simulink model "sldemo_dblcart1"  (R2012b)
settings: Solver=ode23  SolverMode=SingleTasking  StartTime=0  StopTime=250  MaxStep=0.1  RelTol=1e-3  AbsTol=1e-6
PostLoadFcn:
  | crtanim2([],[],[],0,1);
model workspace (MAT data in the model file):
  ka = 1
  m1 = 1
  m2 = 1
  K = [3.08189689488 2.48269889228 0.0803807652926 3.18658131281]
  ae = [0  1  -31.4507297013  0; -1  0  44.8536687603  0; 0  0  -46.6599405981  1; 1  0  -89.5750283103  0]
  be = [0  31.4507297013; 1  -43.8536687603; 0  46.6599405981; 0  88.5750283103]
  ce = [1  0  0  0; 0  1  0  0; 0  0  1  0; 0  0  0  1]
  de = [0  0; 0  0; 0  0; 0  0]
  xSpr = [0; 0.4; 0.8; 1.6; 2.4; 3.2; 3.6; 4]
  xBx1 = [0; 0; -2; -2; 0]
  xBx2 = [0; 2; 2; 0; 0]
Description:
  | Double Spring Mass System
  | 
  | This example shows how to model a double spring-mass-damper system with a periodically
  | varying forcing function.  Associated with the example is an animation function
  | that will automatically open a figure window and display to it. In this system,
  | the only sensor is attached to the mass on the left, and the actuator is
  | attached to the mass on the left. State estimation and LQR control are used.
settings Model: ExtModeAutoUpdateStatusClock=off  Creator=The MathWorks Inc.  LastModifiedBy=re40768
settings DataIOCC: ExternalInput=[]  InitialState=[]  LimitDataPoints=off  SignalLoggingSaveFormat=ModelDataLogs  SaveOutput=off  SaveTime=off
settings OptimizationCC: BlockReduction=off  BooleanDataType=off  InlineInvariantSignals=on  InitFltsAndDblsToZero=on  BufferReusableBoundary=off
settings DebuggingCC: SaveWithParameterizedLinksMsg=none  SignalResolutionControl=TryResolveAllWithWarning  SolverPrmCheckMsg=none  MultiTaskDSMMsg=warning  MultiTaskCondExecSysMsg=none  FcnCallInpInsideContextMsg=UseLocalSettings  BusObjectLabelMismatch=none
settings HardwareCC: TargetUnknown=on
settings RTWCC: IncludeERTFirstTime=on
settings GRTTargetCC: TargetFcnLib=ansi_tfl_tmw.mat  CombineOutputUpdateFcns=off  GRTInterface=on

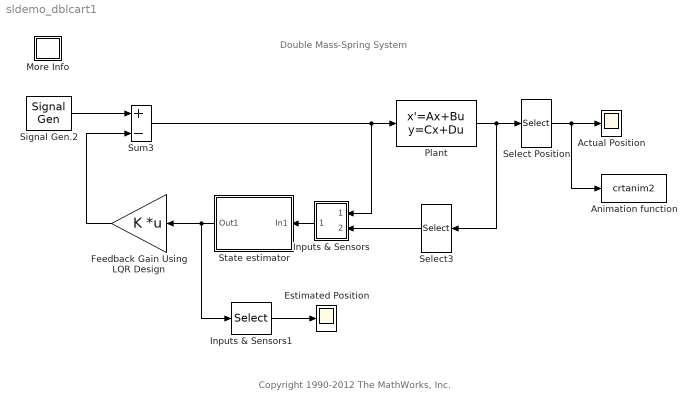
== system sldemo_dblcart1 ==
  note: Double Mass-Spring System
  note: Copyright 1990-2012 The MathWorks, Inc.
  Actual Position : Scope
      settings: TickLabels=on  TimeRange=40.000000
  Animation function : S-Function  FunctionName=crtanim2  Parameters=0.1  EnableBusSupport=off
      settings: DeleteFcn=shh = get(0,'ShowHiddenHandles');set(0,'ShowHiddenHandles','on');if ~isempty(findobj('type','figure','name','dblcart1 Animation'));close('dblcart1 Animation'); end;set(0,'ShowHiddenHandles',shh);
  Estimated Position : Scope
      settings: TickLabels=on  TimeRange=40.000000
  Feedback Gain Using LQR Design : Gain  Gain=K  Multiplication=Matrix(K*u) (u vector)
  Inputs & Sensors : Subsystem
  Inputs & Sensors1 : Selector  InputPortWidth=4  IndexOptions=Index vector (dialog)  Indices=[1 3]  OutputSizes=1
  More Info : Subsystem
      settings: OpenFcn=showdemo(bdroot(gcs))
      mask Display: disp('?')
  Plant : StateSpace  A=[0 1 0 0; -ka/m1 0 ka/m1 0; 0 0 0 1;ka/m2 0 -ka/m2 0]  B=[0; 1; 0; 0]  C=[1 0 0 0;0 0 1 0;0 0 1 0]  D=zeros(3,1)
  Select Position : Selector  InputPortWidth=3  IndexOptions=Index vector (dialog)  Indices=[1,2]  OutputSizes=1
  Select3 : Selector  InputPortWidth=3  IndexOptions=Index vector (dialog)  Indices=3  OutputSizes=1
  Signal Gen.2 : SignalGenerator  WaveForm=square  Amplitude=15  Frequency=0.300000  Units=rad/sec
  State estimator : Subsystem
  Sum3 : Sum  Inputs=+-  SaturateOnIntegerOverflow=on  InputSameDT=on  OutDataTypeStr=Inherit: Same as first input
  wires:
  State estimator/1(Out1) -> Inputs & Sensors1/1, Feedback Gain Using LQR Design/1
  Inputs & Sensors/1(Out1) -> State estimator/1(In1)
  Sum3/1 -> Inputs & Sensors/1(In1), Plant/1
  Feedback Gain Using LQR Design/1 -> Sum3/2
  Plant/1 -> Select3/1, Select Position/1
  Signal Gen.2/1 -> Sum3/1
  Inputs & Sensors1/1 -> Estimated Position/1
  Select3/1 -> Inputs & Sensors/2(In2)
  Select Position/1 -> Actual Position/1, Animation function/1

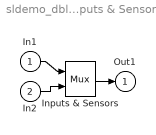
== system sldemo_dblcart1/Inputs & Sensors ==
  In1 : Inport
  In2 : Inport  Port=2
  Inputs & Sensors : Mux  Inputs=2
  Out1 : Outport  InitialOutput=0
  wires:
  In1/1 -> Inputs & Sensors/1
  In2/1 -> Inputs & Sensors/2
  Inputs & Sensors/1 -> Out1/1

== system sldemo_dblcart1/More Info ==

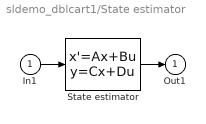
== system sldemo_dblcart1/State estimator ==
  In1 : Inport
  State estimator : StateSpace  A=ae  B=be  C=ce  D=de
  Out1 : Outport  InitialOutput=0
  wires:
  In1/1 -> State estimator/1
  State estimator/1 -> Out1/1
